simulink model "p_c_v1"  (R2014b)
settings: Solver=ode3  StartTime=0.0  StopTime=simtime  FixedStep=0.001  RelTol=1e-3
values from neighbouring files (symbols this model uses):
  a = 1    [path_config_cos.m]    (also in path_planning.m; path_planning_v0.m; path_planning_v1.m; path_planning_v2.m = 0.5)
  b = -1.5    [path_planning.m]    (also in path_planning_v1.m = 0; path_planning_v2.m = 0; run.m = -1; run_abg.m = 0)
  init_state = [init_x_c;init_theta]    [path_planning_v0.m]    (also in path_planning_v1.m; path_planning_v2.m; run.m = [-5;pi]; run_visual.m = [-5;pi])
  init_state_dot = [0;0]    [path_planning_v0.m]    (also in path_planning_v1.m; path_planning_v2.m; run.m; run_visual.m)
  init_x_p = -9    [path_planning.m]    (also in path_planning_v0.m = -5; path_planning_v1.m = -6; path_planning_v2.m = 1; run.m = -5)
  init_x_p_dot = 0    [path_planning.m]    (also in path_planning_v0.m = 1; path_planning_v1.m = 10; path_planning_v2.m = 10; run.m)
  p = 0    [path_planning_v1.m]    (also in path_planning_v2.m = -2.5; run_abg.m; run_alpha.m = -2.5)
  w = pi/5    (= 0.628318530718)    [path_config_cos.m]    (also in path_planning.m; path_planning_v0.m; path_planning_v1.m; path_planning_v2.m = 0.314159265359)
settings Model: Creator=Fredrik  LastModifiedBy=Fredrik

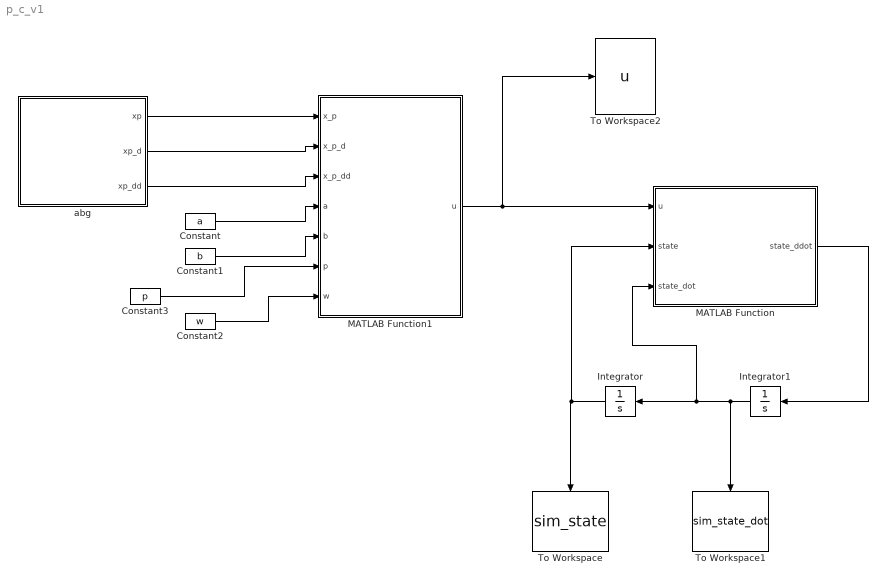
== system p_c_v1 ==
  Constant : Constant  Value=a
  Constant1 : Constant  Value=b
  Constant2 : Constant  Value=w
  Constant3 : Constant  Value=p
  Integrator : Integrator  InitialCondition=init_state
  Integrator1 : Integrator  InitialCondition=init_state_dot
  MATLAB Function : MATLAB Function  TreatAsAtomicUnit=on
  MATLAB Function1 : MATLAB Function  TreatAsAtomicUnit=on
  To Workspace : ToWorkspace  VariableName=sim_state  SaveFormat=Structure With Time  SampleTime=-1
  To Workspace1 : ToWorkspace  VariableName=sim_state_dot  SaveFormat=Structure With Time  SampleTime=-1
  To Workspace2 : ToWorkspace  VariableName=u  SaveFormat=Structure With Time  SampleTime=-1
  abg : Subsystem
  wires:
  MATLAB Function/1(state_ddot) -> Integrator1/1
  Integrator1/1 -> Integrator/1, MATLAB Function/3(state_dot), To Workspace1/1
  Integrator/1 -> To Workspace/1, MATLAB Function/2(state)
  Constant/1 -> MATLAB Function1/4(a)
  Constant1/1 -> MATLAB Function1/5(b)
  Constant2/1 -> MATLAB Function1/7(w)
  abg/1(xp) -> MATLAB Function1/1(x_p)
  abg/2(xp_d) -> MATLAB Function1/2(x_p_d)
  abg/3(xp_dd) -> MATLAB Function1/3(x_p_dd)
  MATLAB Function1/1(u) -> MATLAB Function/1(u), To Workspace2/1
  Constant3/1 -> MATLAB Function1/6(p)

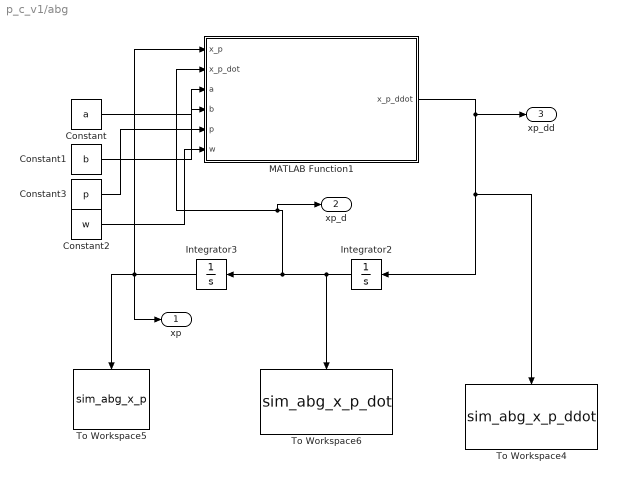
== system p_c_v1/abg ==
  Constant : Constant  Value=a
  Constant1 : Constant  Value=b
  Constant2 : Constant  Value=w
  Constant3 : Constant  Value=p
  Integrator2 : Integrator  InitialCondition=init_x_p_dot
  Integrator3 : Integrator  InitialCondition=init_x_p
  MATLAB Function1 : MATLAB Function  TreatAsAtomicUnit=on
  To Workspace4 : ToWorkspace  VariableName=sim_abg_x_p_ddot  SaveFormat=Structure With Time  SampleTime=-1
  To Workspace5 : ToWorkspace  VariableName=sim_abg_x_p  SaveFormat=Structure With Time  SampleTime=-1
  To Workspace6 : ToWorkspace  VariableName=sim_abg_x_p_dot  SaveFormat=Structure With Time  SampleTime=-1
  xp : Outport
  xp_d : Outport  Port=2
  xp_dd : Outport  Port=3
  wires:
  Integrator3/1 -> xp/1, MATLAB Function1/1(x_p), To Workspace5/1
  MATLAB Function1/1(x_p_ddot) -> xp_dd/1, To Workspace4/1, Integrator2/1
  Constant2/1 -> MATLAB Function1/6(w)
  Constant1/1 -> MATLAB Function1/4(b)
  Constant/1 -> MATLAB Function1/3(a)
  Integrator2/1 -> To Workspace6/1, xp_d/1, MATLAB Function1/2(x_p_dot), Integrator3/1
  Constant3/1 -> MATLAB Function1/5(p)

== matlab function p_c_v1/abg/MATLAB Function1 ==
  data: x_p input; x_p_ddot output; x_p_dot input; a input; b input; p input; w input
function x_p_ddot  = fcn(x_p, x_p_dot,a,b,p,w)
%#codegen

g=9.81;

% cos param v1

alfa = (1+(a*cos(w*x_p+p)+b)*a*sin(w*x_p+p)*w/sqrt(1-(a*cos(w*x_p+p)+b)^2))*(a*cos(w*x_p+p)+b)-(a*cos(w*x_p+p)+b)*a*sin(w*x_p+p)*w/(sqrt(1-(a*cos(w*x_p+p)+b)^2)*sqrt((a*cos(w*x_p+p)+b)^2));
beta = (-(a*cos(w*x_p+p)+b)^2*a^2*sin(w*x_p+p)^2*w^2/(1-(a*cos(w*x_p+p)+b)^2)^(3/2)-a^2*sin(w*x_p+p)^2*w^2/sqrt(1-(a*cos(w*x_p+p)+b)^2)+(a*cos(w*x_p+p)+b)*a*cos(w*x_p+p)*w^2/sqrt(1-(a*cos(w*x_p+p)+b)^2))*(a*cos(w*x_p+p)+b)+(a*cos(w*x_p+p)+b)^2*a^2*sin(w*x_p+p)^2*w^2/((1-(a*cos(w*x_p+p)+b)^2)^(3/2)*sqrt((a*cos(w*x_p+p)+b)^2))+a^2*sin(w*x_p+p)^2*w^2/(sqrt(1-(a*cos(w*x_p+p)+b)^2)*sqrt((a*cos(w*x_p+p)+b)^2))-(a*cos(w*x_p+p)+b)*a*cos(w*x_p+p)*w^2/(sqrt(1-(a*cos(w*x_p+p)+b)^2)*sqrt((a*cos(w*x_p+p)+b)^2))-(a*cos(w*x_p+p)+b)^2*a^2*sin(w*x_p+p)^2*w^2/(sqrt(1-(a*cos(w*x_p+p)+b)^2)*((a*cos(w*x_p+p)+b)^2)^(3/2));
gamma = g*sqrt(1-(a*cos(w*x_p+p)+b)^2);




x_p_ddot = (-beta*(x_p_dot^2) - gamma)/alfa;

== matlab function p_c_v1/MATLAB Function ==
  data: u input; state_ddot output size=2; state input size=2; state_dot input size=2
function state_ddot  = fcn(u,state, state_dot)



x = state(1);
theta = state(2);
x_dot = state_dot(1);
theta_dot = state_dot(2);
g = 9.81;



x_ddot = (1/(cos(theta)^2-2))*(g*sin(theta)*cos(theta) - u - sin(theta)*theta_dot^2);
theta_ddot = (1/(cos(theta)^2-2))*(-2*g*sin(theta) + u*cos(theta) + sin(theta)*cos(theta)*theta_dot^2);


state_ddot = [x_ddot; theta_ddot];

== matlab function p_c_v1/MATLAB Function1 ==
  data: u output; x_p input; x_p_d input; x_p_dd input; a input; b input; p input; w input
function u = fcn(x_p, x_p_d, x_p_dd, a, b,p,w)
%#codegen

g=9.81;




%cos param v1

x_c_dd = (1+(a*cos(w*x_p+p)+b)*a*sin(w*x_p+p)*w/sqrt(1-(a*cos(w*x_p+p)+b)^2))*(x_p_dd)+(-(a*cos(w*x_p+p)+b)^2*a^2*sin(w*x_p+p)^2*w^2/(1-(a*cos(w*x_p+p)+b)^2)^(3/2)-a^2*sin(w*x_p+p)^2*w^2/sqrt(1-(a*cos(w*x_p+p)+b)^2)+(a*cos(w*x_p+p)+b)*a*cos(w*x_p+p)*w^2/sqrt(1-(a*cos(w*x_p+p)+b)^2))*(x_p_d)^2;
theta_d = -(a*cos(w*x_p+p)+b)*a*sin(w*x_p+p)*w*(x_p_d)/(sqrt(1-(a*cos(w*x_p+p)+b)^2)*sqrt((a*cos(w*x_p+p)+b)^2));
theta_dd = ((a*cos(w*x_p+p)+b)^2*a^2*sin(w*x_p+p)^2*w^2/((1-(a*cos(w*x_p+p)+b)^2)^(3/2)*sqrt((a*cos(w*x_p+p)+b)^2))+a^2*sin(w*x_p+p)^2*w^2/(sqrt(1-(a*cos(w*x_p+p)+b)^2)*sqrt((a*cos(w*x_p+p)+b)^2))-(a*cos(w*x_p+p)+b)*a*cos(w*x_p+p)*w^2/(sqrt(1-(a*cos(w*x_p+p)+b)^2)*sqrt((a*cos(w*x_p+p)+b)^2))-(a*cos(w*x_p+p)+b)^2*a^2*sin(w*x_p+p)^2*w^2/(sqrt(1-(a*cos(w*x_p+p)+b)^2)*((a*cos(w*x_p+p)+b)^2)^(3/2)))*(x_p_d)^2-(a*cos(w*x_p+p)+b)*a*sin(w*x_p+p)*w*(x_p_dd)/(sqrt(1-(a*cos(w*x_p+p)+b)^2)*sqrt((a*cos(w*x_p+p)+b)^2));

ss = -sqrt(1-(a*cos(w*x_p+p)+b)^2);
cc = a*cos(w*x_p+p)+b;




u = ( 2*x_c_dd + cc*theta_dd - ss*(theta_d^2) );
